simulink model "GA_PID_sim"  (R2023a)
settings: Solver=VariableStepAuto  StartTime=0.0  StopTime=tsim  RelTol=1e-3
undefined symbols (not defined in the file or in its folder): Ktest
settings Model: Creator=luand  LastModifiedBy=luand
settings DataIOCC: ReturnWorkspaceOutputs=off

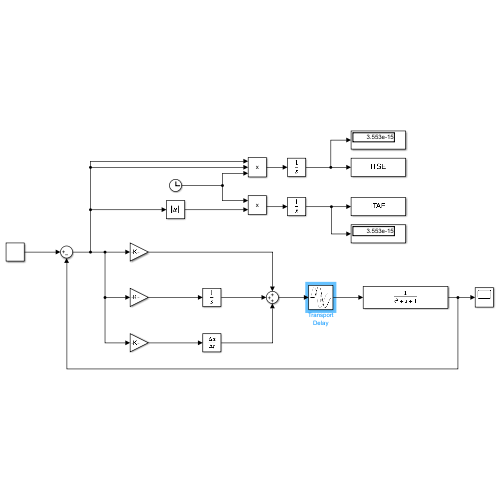
[thumbnail: Simulink's stored preview of the top-level diagram]
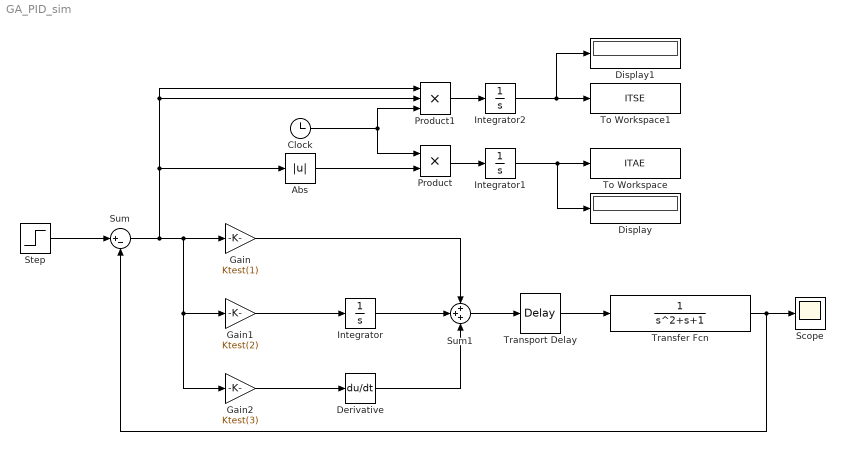
== system GA_PID_sim ==
  Abs : Abs  SaturateOnIntegerOverflow=off
  Clock : Clock
  Derivative : Derivative
  Display : Display
  Display1 : Display
  Gain : Gain  Gain=Ktest(1)
  Gain1 : Gain  Gain=Ktest(2)
  Gain2 : Gain  Gain=Ktest(3)
  Integrator : Integrator
  Integrator1 : Integrator
  Integrator2 : Integrator
  Product : Product
  Product1 : Product  Inputs=3
  Scope : Scope
  Step : Step  SampleTime=0
  Sum : Sum  Inputs=|+-
  Sum1 : Sum  Inputs=+++
  To Workspace : ToWorkspace  VariableName=ITAE  SampleTime=-1
  To Workspace1 : ToWorkspace  VariableName=ITSE  SampleTime=-1
  Transfer Fcn : TransferFcn  Denominator=[1 1 1]
  Transport Delay : TransportDelay
  wires:
  Step/1 -> Sum/1
  Sum/1 -> Product1/2, Product1/1, Abs/1, Gain2/1, Gain1/1, Gain/1
  Gain1/1 -> Integrator/1
  Gain2/1 -> Derivative/1
  Gain/1 -> Sum1/1
  Integrator/1 -> Sum1/2
  Derivative/1 -> Sum1/3
  Sum1/1 -> Transport Delay/1
  Transfer Fcn/1 -> Sum/2, Scope/1
  Clock/1 -> Product/1, Product1/3
  Abs/1 -> Product/2
  Product/1 -> Integrator1/1
  Transport Delay/1 -> Transfer Fcn/1
  Integrator1/1 -> Display/1, To Workspace/1
  Product1/1 -> Integrator2/1
  Integrator2/1 -> Display1/1, To Workspace1/1
